simulink model "lqr_obs_ref_feed"  (R2023b)
settings: Solver=FixedStepAuto  StartTime=0.0  StopTime=SIMTIME  FixedStep=SIMSTEP  RelTol=1e-3
undefined symbols (not defined in the file): A, B, bias, Bv, C, K, L, N, ref, wave_ampl, wave_length, x0, x0_est
settings Model: Creator=X20  LastModifiedBy=Lorenzo-Desk
settings DataIOCC: ReturnWorkspaceOutputs=off

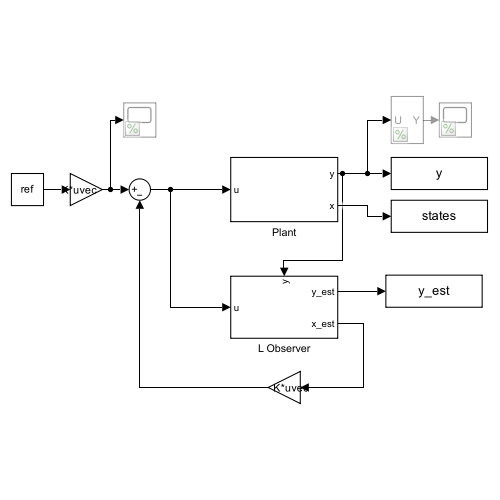
[thumbnail: Simulink's stored preview of the top-level diagram]
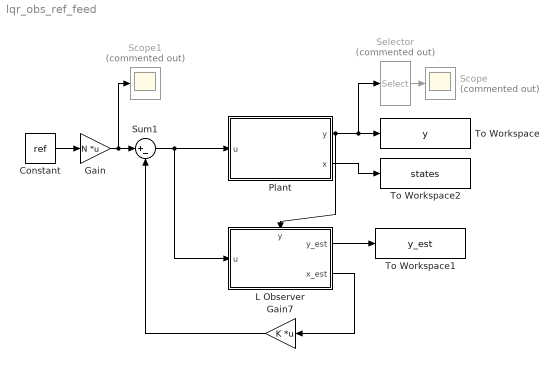
== system lqr_obs_ref_feed ==
  Constant : Constant  Value=ref
  Gain : Gain  Gain=N  Multiplication=Matrix(K*u) (u vector)
  Gain7 : Gain  Gain=K  Multiplication=Matrix(K*u) (u vector)
  L Observer : Subsystem
      settings: PortSchema="{\"entries\":[{\"content\":{\"sides\":[{\"content\":{\"connectorIds\":[\"In1\"]},\"type\":\"ConnectorPlacement.EquallySpacedRectSide\",\"uuid\":\"33578862-1fa2-4e04-9d21-120a6abdc4f0\"},{\"content\":{\"connectorIds\":[\"Out1\",\"Out2\"],\"side\":\"RIGHT\"},\"type\":\"ConnectorPlacement.EquallySpacedRectSide\",\"uuid\":\"7eb22dcc-5863-4bef-ae25-27f07c61a41f\"},{\"content\":{\"connectorIds\":[\"In2\"],\"side\":\"TOP\"},\"type\":\"ConnectorPlacement.EquallySpacedRectSide\",\"uuid\":\"2c4617ba-ebd3-4081-ad3f-53dcb79a95a9\"}]},\"type\":\"ConnectorPlacement.EquallySpacedConnector\",\"uuid\":\"5c678615-8861-4259-9d7f-3a4f22b844ca\"}],\"packageUris\":[\"http://schema.mathworks.com/mf0/Connector/R2020b\"],\"version\":\"1.0\"}"
  Plant : Subsystem
  Scope : Scope  Commented=on
  Scope1 : Scope  Commented=on
  Selector : Selector  Commented=on  InputPortWidth=9  IndexOptions=Index vector (dialog)  Indices=[1 2 3]  OutputSizes=1
  Sum1 : Sum  Inputs=|+-
  To Workspace : ToWorkspace  VariableName=y  SaveFormat=Timeseries  SampleTime=-1
  To Workspace1 : ToWorkspace  VariableName=y_est  SaveFormat=Timeseries  SampleTime=-1
  To Workspace2 : ToWorkspace  VariableName=states  SaveFormat=Timeseries  SampleTime=-1
  wires:
  Constant/1 -> Gain/1
  Gain7/1 -> Sum1/2
  Plant/1(y) -> L Observer/2(y), To Workspace/1, Selector/1
  Sum1/1 -> L Observer/1(u), Plant/1(u)
  Selector/1 -> Scope/1
  Gain/1 -> Scope1/1, Sum1/1
  L Observer/1(y_est) -> To Workspace1/1
  L Observer/2(x_est) -> Gain7/1
  Plant/2(x) -> To Workspace2/1

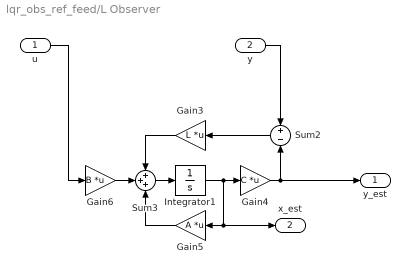
== system lqr_obs_ref_feed/L Observer ==
  u : Inport
  y : Inport  Port=2
  Gain3 : Gain  Gain=L  Multiplication=Matrix(K*u) (u vector)
  Gain4 : Gain  Gain=C  Multiplication=Matrix(K*u) (u vector)
  Gain5 : Gain  Gain=A  Multiplication=Matrix(K*u) (u vector)
  Gain6 : Gain  Gain=B  Multiplication=Matrix(K*u) (u vector)
  Integrator1 : Integrator  InitialCondition=x0_est
  Sum2 : Sum  Inputs=+|-
  Sum3 : Sum  Inputs=+++
  y_est : Outport
  x_est : Outport  Port=2
  wires:
  Gain4/1 -> y_est/1, Sum2/2
  Integrator1/1 -> Gain4/1, Gain5/1, x_est/1
  u/1 -> Gain6/1
  Sum2/1 -> Gain3/1
  Gain3/1 -> Sum3/1
  Gain6/1 -> Sum3/2
  Gain5/1 -> Sum3/3
  Sum3/1 -> Integrator1/1
  y/1 -> Sum2/1

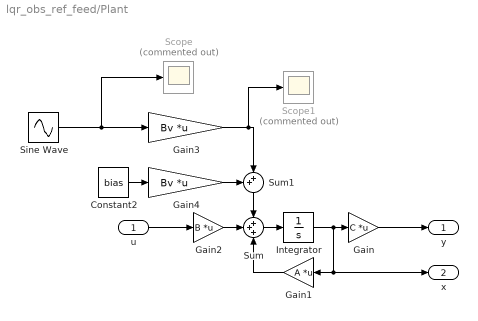
== system lqr_obs_ref_feed/Plant ==
  u : Inport
  Constant2 : Constant  Value=bias
  Gain : Gain  Gain=C  Multiplication=Matrix(K*u) (u vector)
  Gain1 : Gain  Gain=A  Multiplication=Matrix(K*u) (u vector)
  Gain2 : Gain  Gain=B  Multiplication=Matrix(K*u) (u vector)
  Gain3 : Gain  Gain=Bv  Multiplication=Matrix(K*u) (u vector)
  Gain4 : Gain  Gain=Bv  Multiplication=Matrix(K*u) (u vector)
  Integrator : Integrator  InitialCondition=x0
  Scope : Scope  Commented=on
  Scope1 : Scope  Commented=on
  Sine Wave : Sin  Amplitude=wave_ampl  Frequency=1./wave_length  SampleTime=0
  Sum : Sum  Inputs=+++
  Sum1 : Sum  Inputs=++|
  y : Outport
  x : Outport  Port=2
  wires:
  Gain/1 -> y/1
  u/1 -> Gain2/1
  Sum/1 -> Integrator/1
  Integrator/1 -> Gain/1, x/1, Gain1/1
  Gain1/1 -> Sum/3
  Gain2/1 -> Sum/2
  Sum1/1 -> Sum/1
  Gain4/1 -> Sum1/1
  Constant2/1 -> Gain4/1
  Gain3/1 -> Scope1/1, Sum1/2
  Sine Wave/1 -> Scope/1, Gain3/1
